simulink subsystem "lqr_controller"  (R2025a)
settings: Solver=VariableStepAuto  StartTime=0.0  StopTime=10.0  RelTol=1e-3
undefined symbols (not defined in the file or in its folder): Ki, Kp
settings Model: Creator=johnpye  LastModifiedBy=johnpye

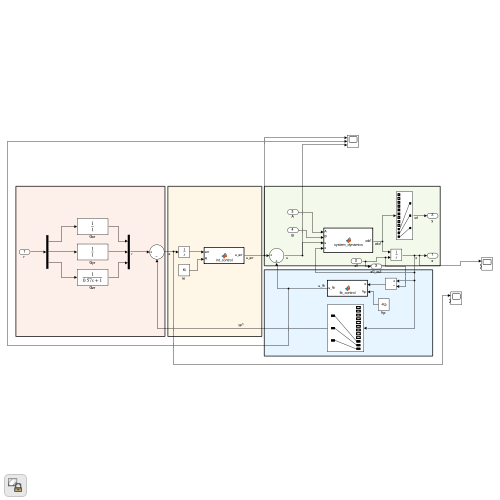
[thumbnail: Simulink's stored preview of the top-level diagram]
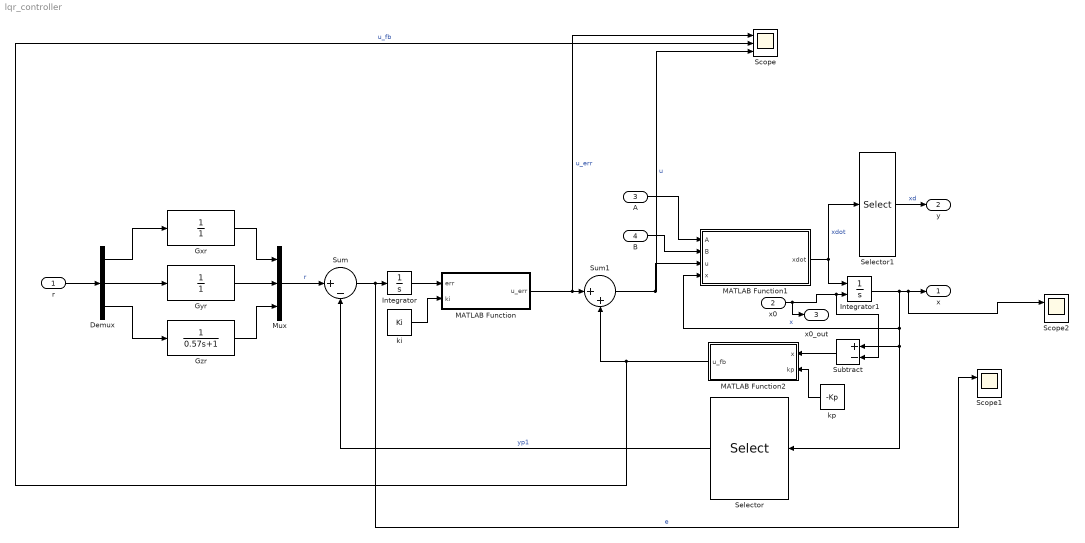
== system lqr_controller ==
  r : Inport
  x0 : Inport  Port=2
  A : Inport  Port=3
  B : Inport  Port=4
  Demux : Demux  Outputs=3
  Gxr : TransferFcn  Denominator=[1]
  Gyr : TransferFcn  Denominator=[1]
  Gzr : TransferFcn  Denominator=[0.57 1]
  Integrator : Integrator
  Integrator1 : Integrator  InitialConditionSource=external  InitialCondition=[0; 0; 0; 0; 0; 0; 0; 0; 0; -1; 0; 0]
  MATLAB Function : MATLAB Function  TreatAsAtomicUnit=on
  MATLAB Function1 : MATLAB Function  TreatAsAtomicUnit=on
  MATLAB Function2 : MATLAB Function  TreatAsAtomicUnit=on
  Mux : Mux  Inputs=3
  Scope : Scope  NumInputPorts=3
      settings: ActiveDisplayYMinimum=-1.0009054081910192E+10  ActiveDisplayYMaximum=1.3756629951484056E+9  DataLoggingVariableName=ScopeData21
  Scope1 : Scope  NumInputPorts=2
      settings: ActiveDisplayYMinimum=-385.13541358093136  ActiveDisplayYMaximum=43.626670712045829  DataLoggingVariableName=ScopeData22
  Scope2 : Scope  NumInputPorts=2
      settings: ActiveDisplayYMinimum=-343.67829957617272  ActiveDisplayYMaximum=604.98039344378071  DataLoggingVariableName=ScopeData24
  Selector : Selector  InputPortWidth=12  IndexOptions=Index vector (dialog)  Indices=[10 11 12]  OutputSizes=1
  Selector1 : Selector  InputPortWidth=12  IndexOptions=Index vector (dialog)  Indices=[10 11 12]  OutputSizes=1
  Subtract : Sum  Inputs=+-
  Sum : Sum  Inputs=|+-
  Sum1 : Sum  Inputs=|++
  ki : Constant  Value=Ki
  kp : Constant  Value=-Kp
  x : Outport
  y : Outport  Port=2
  x0_out : Outport  Port=3
  wires:
  r/1 -> Demux/1
  Demux/1 -> Gxr/1
  Demux/2 -> Gyr/1
  Demux/3 -> Gzr/1
  Gxr/1 -> Mux/1
  Gyr/1 -> Mux/2
  Gzr/1 -> Mux/3
  Mux/1 -> Sum/1  "r"
  Sum/1 -> Integrator/1, Scope1/1  "e"
  Integrator/1 -> MATLAB Function/1(err)
  ki/1 -> MATLAB Function/2(ki)
  Sum1/1 -> MATLAB Function1/3(u), Scope/3  "u"
  A/1 -> MATLAB Function1/1(A)
  B/1 -> MATLAB Function1/2(B)
  MATLAB Function1/1(xdot) -> Integrator1/1, Selector1/1  "xdot"
  Integrator1/1 -> Selector/1, Subtract/1, MATLAB Function1/4(x), x/1, Scope2/1  "x"
  MATLAB Function2/1(u_fb) -> Sum1/2, Scope/2  "u_fb"
  Selector/1 -> Sum/2  "yp1"
  kp/1 -> MATLAB Function2/2(kp)
  x0/1 -> Integrator1/2, Subtract/2, x0_out/1
  Selector1/1 -> y/1  "xd"
  Subtract/1 -> MATLAB Function2/1(x)
  MATLAB Function/1(u_err) -> Sum1/1, Scope/1  "u_err"

== matlab function lqr_controller/MATLAB Function ==
  data: err input; u_err output; ki input
function u_err = int_control(err, ki)

err = reshape(err, [3, 1]);
u_err = ki * err;

== matlab function lqr_controller/MATLAB Function1 ==
  data: A input; B input; u input; x input; xdot output
function xdot = system_dynamics(A, B, u, x)

g = 9.81; % m/s^2
l = 0.2; % m
Jmp = 0;
Jxx = 1.8e-3; % kgm^2
Jyy = 1.8e-3; % kgm^2
Jzz = 1.5e-3; % kgm^2
kmt = 0.1; % m

K = B(4,2)*Jxx;
m = (1/B(3,1)) * -K;

u = reshape(u, [4, 1]);
% u(1) = u(1) - 9.81*0.8;
x = reshape(x, [12, 1]);
% xdot = A*x + B*u;
xdot=zeros(12,1);

vx = x(1);
vy = x(2);
vz = x(3);
wx = x(4);
wy = x(5);
wz = x(6);
theta = x(7);
phi = x(8);
psi = x(9);
x = x(10);
T = u(1);
Mx = u(2);
My = u(3);
Mz = u(4);

% Step 3: Calculate derivatives
xdot(1)         = -vz*wy + vy*wz - g*sin(theta);
xdot(2)         = -vx*wz + vz*wx + g*cos(theta)*sin(phi);
xdot(3)         = -vy*wx + vx*wy + g*cos(theta)*cos(phi) - T/m;
xdot(4)         = (1/Jxx)*(-wy*wz*(Jzz - Jyy) + Mx);
xdot(5)         = (1/Jyy)*(-wx*wz*(Jxx - Jzz) + My);
xdot(6)         = Mz / Jzz;
xdot(7)         = wy*cos(phi) - wz*sin(phi);
xdot(8)         = wx + wy*sin(phi)*tan(theta) + wz*cos(phi)*tan(theta);
xdot(9)         = wy*(sin(phi)/cos(theta)) + wz*(cos(phi)/cos(theta));
xdot(10)        = vx*cos(psi)*cos(theta) + ...
                    vy*(-sin(psi)*cos(phi) + cos(psi)*sin(theta)*sin(phi)) + ...
                    vz*(sin(psi)*sin(phi) + cos(psi)*sin(theta)*cos(phi));
xdot(11)        = vx*sin(psi)*cos(theta) + ...
                    vy*(cos(psi)*cos(phi) + sin(psi)*sin(theta)*sin(phi)) + ...
                    vz*(-cos(psi)*sin(phi) + sin(psi)*sin(theta)*cos(phi));
xdot(12)        = vx*sin(theta) - vy*cos(theta)*sin(phi) - vz*cos(theta)*cos(phi);

== matlab function lqr_controller/MATLAB Function2 ==
  data: x input; u_fb output; kp input
function u_fb = fb_control(x, kp)

x = reshape(x, [12, 1]);
u_fb = kp * x;
